simulink model "Fig_7_8__extflc"  (R2024a)
settings: Solver=VariableStepAuto  StartTime=0.0  StopTime=1  RelTol=1e-3
undefined symbols (not defined in the file): gcbh, Ion, Lithium, sps_rtmsupport
libraries: spsSeriesRLCBranchLib x11, spsThreePhaseVIMeasurementLib x5, slpidlib x5, spsIGBTDiodeLib x4, spsVoltageMeasurementLib x4, spsThreePhaseSeriesRLCBranchLib x4, spsUniversalBridgeLib x3, spsPWMGeneratorDCDCLib x3, spsBreakerLib x3, spsDiodeLib x2, spsabctodq0Lib x2, spsCurrentMeasurementLib x2
(part 2 of 2)

== system Fig_7_8__extflc/EVFCS/Battery charging controller ==
  note: Constant current battery charger control
  Add : Sum  Inputs=+-
  Add1 : Sum  Inputs=+-
  PID Controller1 : slpidlib/PID Controller  Controller=PI  Form=Parallel  TimeDomain=Discrete-time  UseExternalTs=off  SampleTime=-1  IntegratorMethod=Forward Euler  FilterMethod=Forward Euler  ControllerParametersSource=internal  P=5  I=0.0005  UseKiTs=off  D=0  UseExternalDerivativeSource=off  N=100  UseFilter=on  TunerSelectOption=Frequency Response Based  InitialConditionSource=internal  InitialConditionForIntegrator=0  InitialConditionForFilter=0  DifferentiatorICPrevScaledInput=0  ExternalReset=none  TrackingMode=off  Kt=1  LimitOutput=off  SatLimitsSource=internal  UpperSaturationLimit=1  LowerSaturationLimit=0  LinearizeAsGain=on  AntiWindupMode=none  Kb=1  LimitIntegrator=off  UpperIntegratorSaturationLimit=inf  LowerIntegratorSaturationLimit=-inf  POutMin=[]  POutMax=[]  IOutMin=[]  IOutMax=[]  DOutMin=[]  DOutMax=[]  NOutMin=[]  NOutMax=[]  SumOutMin=[]  SumOutMax=[]  SaturationOutMin=[]  SaturationOutMax=[]  PParamMin=[]  PParamMax=[]  IParamMin=[]  IParamMax=[]  DParamMin=[]  DParamMax=[]  NParamMin=[]  NParamMax=[]  KbParamMin=[]  KbParamMax=[]  KtParamMin=[]  KtParamMax=[]  KbOutMin=[]  KbOutMax=[]  KtOutMin=[]  KtOutMax=[]  IntegratorOutMin=[]  IntegratorOutMax=[]  FilterOutMin=[]  FilterOutMax=[]  SumI1OutMin=[]  SumI1OutMax=[]  SumI2OutMin=[]  SumI2OutMax=[]  SumI3OutMin=[]  SumI3OutMax=[]  SumI4OutMin=[]  SumI4OutMax=[]  SumDOutMin=[]  SumDOutMax=[]  DifferentiatorOutMin=[]  DifferentiatorOutMax=[]  FilterDiffOutCoefMin=[]  FilterDiffOutCoefMax=[]  ReciprocalOutMin=[]  ReciprocalOutMax=[]  SumDenOutMin=[]  SumDenOutMax=[]  SumNumOutMin=[]  SumNumOutMax=[]  DivideOutMin=[]  DivideOutMax=[]  UdiffTsProdOutMin=[]  UdiffTsProdOutMax=[]  NTsProdOutMin=[]  NTsProdOutMax=[]  UintegralTsProdOutMin=[]  UintegralTsProdOutMax=[]  UngainTsProdOutMin=[]  UngainTsProdOutMax=[]  ClampingZeroOutDataTypeStr=Inherit: Inherit via back propagation  ClampingZeroOutMin=[]  ClampingZeroOutMax=[]  FilterDenConstantOutDataTypeStr=Inherit: Inherit via back propagation  FilterDenConstantOutMin=[]  FilterDenConstantOutMax=[]  PCopyOutDataTypeStr=Inherit: Inherit via back propagation  PCopyOutMin=[]  PCopyOutMax=[]  NCopyOutDataTypeStr=Inherit: Inherit via back propagation  NCopyOutMin=[]  NCopyOutMax=[]  IntegratorContinuousStateAttributes=''  IntegratorStateMustResolveToSignalObject=off  IntegratorRTWStateStorageClass=Auto  FilterContinuousStateAttributes=''  FilterStateMustResolveToSignalObject=off  FilterRTWStateStorageClass=Auto  ParallelPVariant=InternalParameters  IdealPVariant=Disabled  IVariant=InternalParameters  DVariant=Disabled  IntegratorVariant=Discrete  SatVariant=Disabled  AWVariant=Passthrough  PCopyVariant=Disabled  TRVariant=Disabled  FdbkBlocksVariant=Forward  IdealPFdbkVariant=Disabled  SatFdbkVariant=Disabled  DerivativeFilterVariant=Disabled  NVariant=Disabled  NCopyVariant=Disabled_SignalSpec  FilterICVariant=Disabled  IntegratorICVariant=InternalICs  ExternalResetVariant=Disabled  TRSumVariant=Passthrough  SumFdbkVariant=Disabled  SumVariant=Sum_PI  TsampFilterVariant=InternalTs  TsampNgainVariant=Passthrough  TsampIntegralVariant=Disabled_SignalSpec  ExternalSaturationOutDataTypeStr=Inherit: Same as second input  DerivativeSourceVariant=Disabled
  PID Controller2 : slpidlib/PID Controller  Controller=PI  Form=Parallel  TimeDomain=Discrete-time  UseExternalTs=off  SampleTime=-1  IntegratorMethod=Forward Euler  FilterMethod=Forward Euler  ControllerParametersSource=internal  P=-5  I=-0.0005  UseKiTs=off  D=0  UseExternalDerivativeSource=off  N=100  UseFilter=on  TunerSelectOption=Transfer Function Based (PID Tuner App)  InitialConditionSource=internal  InitialConditionForIntegrator=0  InitialConditionForFilter=0  DifferentiatorICPrevScaledInput=0  ExternalReset=none  TrackingMode=off  Kt=1  LimitOutput=off  SatLimitsSource=internal  UpperSaturationLimit=0  LowerSaturationLimit=-5  LinearizeAsGain=on  AntiWindupMode=none  Kb=1  LimitIntegrator=off  UpperIntegratorSaturationLimit=inf  LowerIntegratorSaturationLimit=-inf  POutMin=[]  POutMax=[]  IOutMin=[]  IOutMax=[]  DOutMin=[]  DOutMax=[]  NOutMin=[]  NOutMax=[]  SumOutMin=[]  SumOutMax=[]  SaturationOutMin=[]  SaturationOutMax=[]  PParamMin=[]  PParamMax=[]  IParamMin=[]  IParamMax=[]  DParamMin=[]  DParamMax=[]  NParamMin=[]  NParamMax=[]  KbParamMin=[]  KbParamMax=[]  KtParamMin=[]  KtParamMax=[]  KbOutMin=[]  KbOutMax=[]  KtOutMin=[]  KtOutMax=[]  IntegratorOutMin=[]  IntegratorOutMax=[]  FilterOutMin=[]  FilterOutMax=[]  SumI1OutMin=[]  SumI1OutMax=[]  SumI2OutMin=[]  SumI2OutMax=[]  SumI3OutMin=[]  SumI3OutMax=[]  SumI4OutMin=[]  SumI4OutMax=[]  SumDOutMin=[]  SumDOutMax=[]  DifferentiatorOutMin=[]  DifferentiatorOutMax=[]  FilterDiffOutCoefMin=[]  FilterDiffOutCoefMax=[]  ReciprocalOutMin=[]  ReciprocalOutMax=[]  SumDenOutMin=[]  SumDenOutMax=[]  SumNumOutMin=[]  SumNumOutMax=[]  DivideOutMin=[]  DivideOutMax=[]  UdiffTsProdOutMin=[]  UdiffTsProdOutMax=[]  NTsProdOutMin=[]  NTsProdOutMax=[]  UintegralTsProdOutMin=[]  UintegralTsProdOutMax=[]  UngainTsProdOutMin=[]  UngainTsProdOutMax=[]  ClampingZeroOutDataTypeStr=Inherit: Inherit via back propagation  ClampingZeroOutMin=[]  ClampingZeroOutMax=[]  FilterDenConstantOutDataTypeStr=Inherit: Inherit via back propagation  FilterDenConstantOutMin=[]  FilterDenConstantOutMax=[]  PCopyOutDataTypeStr=Inherit: Inherit via back propagation  PCopyOutMin=[]  PCopyOutMax=[]  NCopyOutDataTypeStr=Inherit: Inherit via back propagation  NCopyOutMin=[]  NCopyOutMax=[]  IntegratorContinuousStateAttributes=''  IntegratorStateMustResolveToSignalObject=off  IntegratorRTWStateStorageClass=Auto  FilterContinuousStateAttributes=''  FilterStateMustResolveToSignalObject=off  FilterRTWStateStorageClass=Auto  ParallelPVariant=InternalParameters  IdealPVariant=Disabled  IVariant=InternalParameters  DVariant=Disabled  IntegratorVariant=Discrete  SatVariant=Disabled  AWVariant=Passthrough  PCopyVariant=Disabled  TRVariant=Disabled  FdbkBlocksVariant=Forward  IdealPFdbkVariant=Disabled  SatFdbkVariant=Disabled  DerivativeFilterVariant=Disabled  NVariant=Disabled  NCopyVariant=Disabled_SignalSpec  FilterICVariant=Disabled  IntegratorICVariant=InternalICs  ExternalResetVariant=Disabled  TRSumVariant=Passthrough  SumFdbkVariant=Disabled  SumVariant=Sum_PI  TsampFilterVariant=InternalTs  TsampNgainVariant=Passthrough  TsampIntegralVariant=Disabled_SignalSpec  ExternalSaturationOutDataTypeStr=Inherit: Same as second input  DerivativeSourceVariant=Disabled
  PWM Generator (DC-DC)1 : spsPWMGeneratorDCDCLib/PWM Generator (DC-DC)  Fsw=20e3  Ts=50e-6
  Vev_ref : Constant  Value=480
  G : Outport
  wires:
  PWM Generator (DC-DC)1/1 -> G/1
  Add/1 -> PID Controller2/1
  Vev_ref/1 -> Add/1
  [Vev] -> Add/2
  [Iev] -> Add1/2
  PID Controller2/1 -> Add1/1
  Add1/1 -> PID Controller1/1
  PID Controller1/1 -> PWM Generator (DC-DC)1/1

== system Fig_7_8__extflc/Dstatcom/Controller/FLC ==
  error : Inport
  Derivative : Derivative
  Fuzzy Logic Controller : fuzblock/Fuzzy Logic  Controller  FIS=flcabcdef  OutputSampleNumber=2  DataType=double  FuzzifiedInputs=off  RuleFiringStrengths=off  RuleOutputs=off  AggregatedOutputs=off  SimulateUsing=Interpreted execution  OutOfRangeInputValueMessage=none  NoRuleFiredMessage=none  EmptyOutputFuzzySetMessage=none
  Mux : Mux  Inputs=2
  output : Outport
  wires:
  Fuzzy Logic Controller/1 -> output/1
  Mux/1 -> Fuzzy Logic Controller/1
  Derivative/1 -> Mux/2
  error/1 -> Derivative/1, Mux/1

== system Fig_7_8__extflc/Dstatcom/Controller/PI1 ==
  In1 : Inport
  Integrator : Integrator  LimitOutput=on  UpperSaturationLimit=500  LowerSaturationLimit=-500
  Ki : Gain  Gain=1200
  Kp : Gain  Gain=800
  Sum8 : Sum  Inputs=|++
  Out1 : Outport
  wires:
  Ki/1 -> Integrator/1
  Kp/1 -> Sum8/1
  Integrator/1 -> Sum8/2
  In1/1 -> Kp/1, Ki/1
  Sum8/1 -> Out1/1

== system Fig_7_8__extflc/Dstatcom/Controller/RYB - ab ==
  Ilr : Inport
  Ily : Inport  Port=2
  Ilb : Inport  Port=3
  Demux : Demux  Outputs=2
  Gain : Gain  Gain=[1 -0.5 -0.5;0 0.866 -0.866]  Multiplication=Matrix(K*u)
  Mux : Mux  Inputs=3
  a : Outport
  b : Outport  Port=2
  wires:
  Demux/1 -> a/1
  Mux/1 -> Gain/1
  Demux/2 -> b/1
  Ilr/1 -> Mux/1
  Ilb/1 -> Mux/3
  Gain/1 -> Demux/1
  Ily/1 -> Mux/2

== system Fig_7_8__extflc/Dstatcom/Controller/RYB - ab1 ==
  Vgr : Inport
  Vgy : Inport  Port=2
  Vgb : Inport  Port=3
  Demux : Demux  Outputs=2
  Gain : Gain  Gain=[1 -0.5 -0.5;0 0.866 -0.866]  Multiplication=Matrix(K*u)
  Mux : Mux  Inputs=3
  Scope : Scope  NumInputPorts=2
  Va : Outport
  Vb : Outport  Port=2
  wires:
  Demux/1 -> Va/1
  Mux/1 -> Scope/2, Gain/1
  Demux/2 -> Scope/1, Vb/1
  Vgr/1 -> Mux/1
  Vgb/1 -> Mux/3
  Gain/1 -> Demux/1
  Vgy/1 -> Mux/2

== system Fig_7_8__extflc/Dstatcom/Controller/RYB - ab2 ==
  Isr : Inport
  Isy : Inport  Port=2
  Isb : Inport  Port=3
  Demux : Demux  Outputs=2
  Gain : Gain  Gain=[1 -0.5 -0.5;0 0.866 -0.866]  Multiplication=Matrix(K*u)
  Mux : Mux  Inputs=3
  Scope : Scope  NumInputPorts=2
  a : Outport
  b : Outport  Port=2
  wires:
  Demux/1 -> a/1
  Mux/1 -> Scope/2, Gain/1
  Demux/2 -> b/1
  Isr/1 -> Mux/1
  Isb/1 -> Mux/3
  Isy/1 -> Mux/2
  Gain/1 -> Scope/1, Demux/1

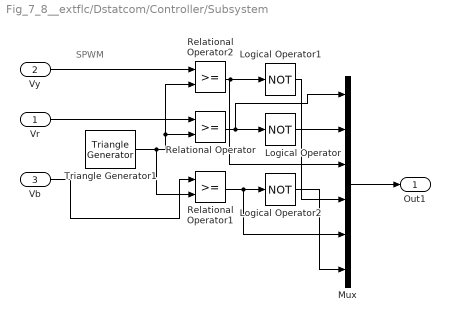
== system Fig_7_8__extflc/Dstatcom/Controller/Subsystem ==
  note: SPWM
  Vr : Inport
  Vy : Inport  Port=2
  Vb : Inport  Port=3
  Logical Operator : Logic  Operator=NOT  IconShape=distinctive  AllPortsSameDT=off  OutDataTypeStr=boolean
  Logical Operator1 : Logic  Operator=NOT  IconShape=distinctive  AllPortsSameDT=off  OutDataTypeStr=boolean
  Logical Operator2 : Logic  Operator=NOT  IconShape=distinctive  AllPortsSameDT=off  OutDataTypeStr=boolean
  Mux : Mux  Inputs=6
  Relational Operator : RelationalOperator  OutDataTypeStr=boolean  InputSameDT=off
  Relational Operator1 : RelationalOperator  OutDataTypeStr=boolean  InputSameDT=off
  Relational Operator2 : RelationalOperator  OutDataTypeStr=boolean  InputSameDT=off
  Triangle Generator1 : spsTriangleGeneratorLib/Triangle Generator  Freq=20e3  Phase=90  Ts=0
  Out1 : Outport
  wires:
  Triangle Generator1/1 -> Relational Operator2/2, Relational Operator/2, Relational Operator1/2
  Relational Operator2/1 -> Mux/3, Logical Operator1/1
  Relational Operator/1 -> Mux/1, Logical Operator/1
  Relational Operator1/1 -> Mux/5, Logical Operator2/1
  Mux/1 -> Out1/1
  Vy/1 -> Relational Operator2/1
  Logical Operator2/1 -> Mux/6
  Logical Operator1/1 -> Mux/4
  Logical Operator/1 -> Mux/2
  Vr/1 -> Relational Operator/1
  Vb/1 -> Relational Operator1/1

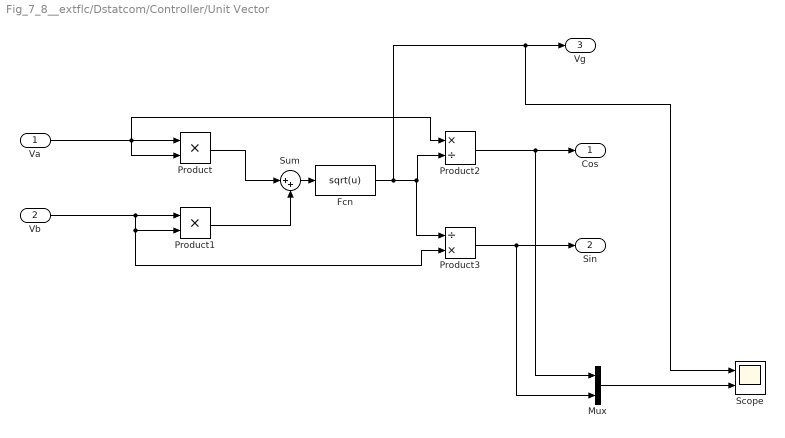
== system Fig_7_8__extflc/Dstatcom/Controller/Unit Vector ==
  Va : Inport
  Vb : Inport  Port=2
  Fcn : Fcn  Expr=sqrt(u)
  Mux : Mux  Inputs=2
  Product : Product
  Product1 : Product
  Product2 : Product  Inputs=*/
  Product3 : Product  Inputs=/*
  Scope : Scope  NumInputPorts=2
  Sum : Sum  Inputs=|++
  Cos : Outport
  Sin : Outport  Port=2
  Vg : Outport  Port=3
  wires:
  Sum/1 -> Fcn/1
  Va/1 -> Product2/1, Product/2, Product/1
  Vb/1 -> Product1/1, Product1/2, Product3/2
  Product/1 -> Sum/1
  Product1/1 -> Sum/2
  Product3/1 -> Mux/2, Sin/1
  Product2/1 -> Mux/1, Cos/1
  Fcn/1 -> Scope/1, Vg/1, Product3/1, Product2/2
  Mux/1 -> Scope/2

== system Fig_7_8__extflc/Dstatcom/Controller/ab - RYB ==
  a : Inport
  b : Inport  Port=2
  Demux : Demux  Outputs=3
  Gain : Gain  Gain=[1 0;-1/2 sqrt(3)/2;-1/2 -sqrt(3)/2]  Multiplication=Matrix(K*u)
  Mux : Mux  Inputs=2
  R : Outport
  Y : Outport  Port=2
  B : Outport  Port=3
  wires:
  b/1 -> Mux/2
  Gain/1 -> Demux/1
  a/1 -> Mux/1
  Demux/2 -> Y/1
  Mux/1 -> Gain/1
  Demux/1 -> R/1
  Demux/3 -> B/1

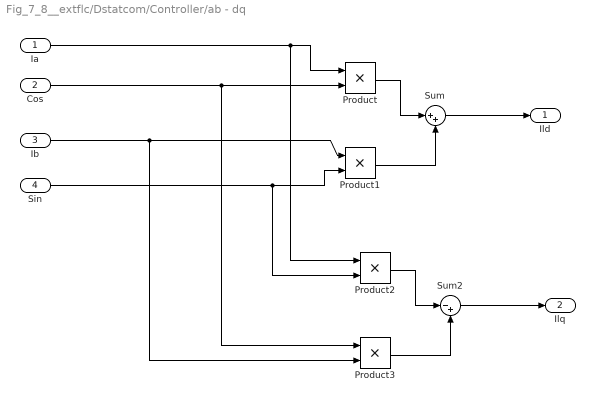
== system Fig_7_8__extflc/Dstatcom/Controller/ab - dq ==
  Ia : Inport
  Cos : Inport  Port=2
  Ib : Inport  Port=3
  Sin : Inport  Port=4
  Product{,1..3} (4 alike) : Product
  Sum : Sum  Inputs=|++
  Sum2 : Sum  Inputs=|-+
  Ild : Outport
  Ilq : Outport  Port=2
  wires:
  Product/1 -> Sum/1
  Sin/1 -> Product2/2, Product1/2
  Product1/1 -> Sum/2
  Ia/1 -> Product2/1, Product/1
  Sum/1 -> Ild/1
  Ib/1 -> Product3/2, Product1/1
  Product2/1 -> Sum2/1
  Product3/1 -> Sum2/2
  Sum2/1 -> Ilq/1
  Cos/1 -> Product3/1, Product/2

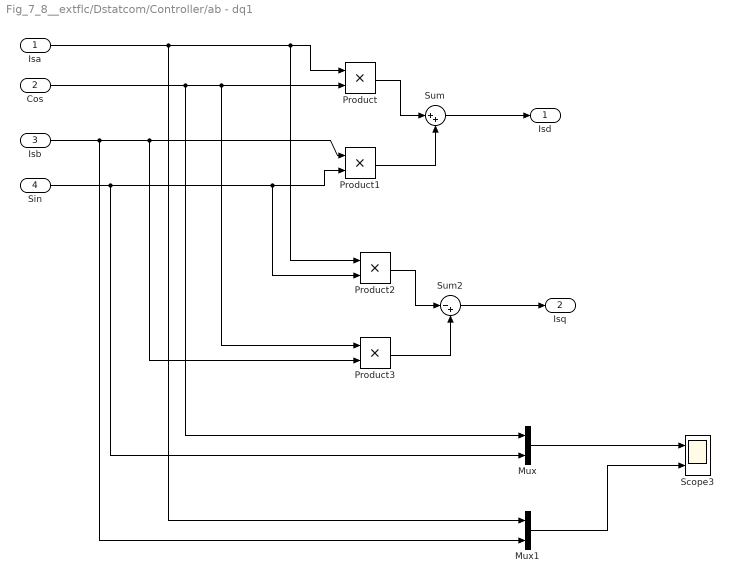
== system Fig_7_8__extflc/Dstatcom/Controller/ab - dq1 ==
  Isa : Inport
  Cos : Inport  Port=2
  Isb : Inport  Port=3
  Sin : Inport  Port=4
  Mux : Mux  Inputs=2
  Mux1 : Mux  Inputs=2
  Product{,1..3} (4 alike) : Product
  Scope3 : Scope  NumInputPorts=2
  Sum : Sum  Inputs=|++
  Sum2 : Sum  Inputs=|-+
  Isd : Outport
  Isq : Outport  Port=2
  wires:
  Product/1 -> Sum/1
  Sin/1 -> Mux/2, Product2/2, Product1/2
  Product1/1 -> Sum/2
  Isa/1 -> Mux1/1, Product2/1, Product/1
  Sum/1 -> Isd/1
  Isb/1 -> Mux1/2, Product3/2, Product1/1
  Product2/1 -> Sum2/1
  Product3/1 -> Sum2/2
  Sum2/1 -> Isq/1
  Cos/1 -> Mux/1, Product3/1, Product/2
  Mux/1 -> Scope3/1
  Mux1/1 -> Scope3/2

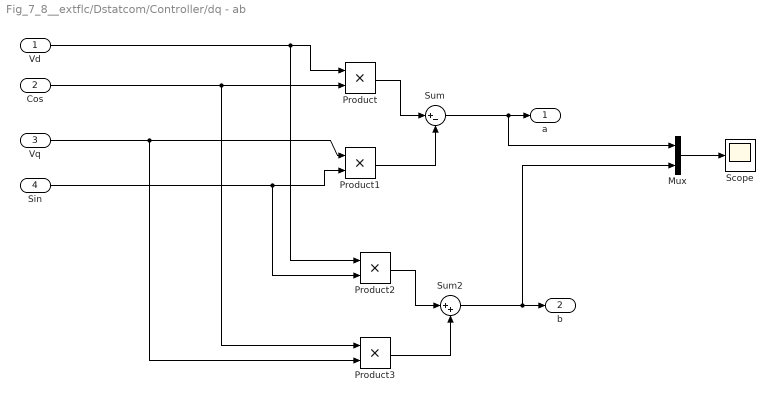
== system Fig_7_8__extflc/Dstatcom/Controller/dq - ab ==
  Vd : Inport
  Cos : Inport  Port=2
  Vq : Inport  Port=3
  Sin : Inport  Port=4
  Mux : Mux  Inputs=2
  Product{,1..3} (4 alike) : Product
  Scope : Scope
  Sum : Sum  Inputs=|+-
  Sum2 : Sum  Inputs=|++
  a : Outport
  b : Outport  Port=2
  wires:
  Cos/1 -> Product/2, Product3/1
  Sum2/1 -> Mux/2, b/1
  Product3/1 -> Sum2/2
  Product2/1 -> Sum2/1
  Vq/1 -> Product1/1, Product3/2
  Sum/1 -> Mux/1, a/1
  Vd/1 -> Product/1, Product2/1
  Product1/1 -> Sum/2
  Sin/1 -> Product1/2, Product2/2
  Product/1 -> Sum/1
  Mux/1 -> Scope/1

== system Fig_7_8__extflc/Dstatcom/D_Statcom/Subsystem ==
  Breaker : spsBreakerLib/Breaker  InitialState=1  SwitchingTimes="[1/60  5/60]"  External=on  BreakerResistance=0.01  SnubberResistance=1e6  SnubberCapacitance=inf  Measurements=None  MoreParameters=on  NoBreakLoop=off
  DC Voltage Source : spsDCVoltageSourceLib/DC Voltage Source  Amplitude=730  Measurements=None
  Series RLC Branch2 : spsSeriesRLCBranchLib/Series RLC Branch  LConnTagsString=__new0  RConnTagsString=__new0  BranchType=R  Resistance=0.001  Inductance=1e-3  SetiL0=off  InitialCurrent=0  Capacitance=1000e-6  Setx0=off  InitialVoltage=0  Measurements=None
  + : PMIOPort  Side=Left
  - : PMIOPort  Port=2  Side=Right
  wires:
  [T24_2155_1229794295581] -> Breaker/1
  connections:
  DC Voltage Source/RConn1 -- Series RLC Branch2/RConn1
  DC Voltage Source/LConn1 -- -/RConn1
  Breaker/LConn1 -- +/RConn1
  Breaker/RConn1 -- Series RLC Branch2/LConn1

== matlab function Fig_7_8__extflc/BOOST CONVERTER/PnO/PERTURB & OBSERVE ALGORITHM ==
  data: Vpv input; D output; Ipv input
function D = PnO(Vpv, Ipv)

persistent Dprev Pprev Vprev

if isempty(Dprev)
    Dprev = 0.7;
    Vprev = 145;
    Pprev = 1000;
end

deltaD = 125e-6

% Caluclate PV Power
Ppv = Vpv*Ipv

% Increase or decrease duty cycle based on conditions
if (Ppv-Pprev) ~= 0
    if (Ppv-Pprev) > 0
        if (Vpv-Vprev) > 0
            D = Dprev - deltaD;
        else
            D = Dprev + deltaD;
        end
    else
        if (Vpv - Vprev) > 0
            D = Dprev + deltaD;
        else
            D = Dprev - deltaD;
        end
    end
else
    D = Dprev;
end

% Update interval values
Dprev = D;
Vprev = Vpv;
Pprev = Ppv;

== matlab function Fig_7_8__extflc/BOOST CONVERTER1/PnO/PERTURB & OBSERVE ALGORITHM ==
  data: Vpv input; D output; Ipv input
function D = PnO(Vpv, Ipv)

persistent Dprev Pprev Vprev

if isempty(Dprev)
    Dprev = 0.7;
    Vprev = 145;
    Pprev = 1000;
end

deltaD = 125e-6

% Caluclate PV Power
Ppv = Vpv*Ipv

% Increase or decrease duty cycle based on conditions
if (Ppv-Pprev) ~= 0
    if (Ppv-Pprev) > 0
        if (Vpv-Vprev) > 0
            D = Dprev - deltaD;
        else
            D = Dprev + deltaD;
        end
    else
        if (Vpv - Vprev) > 0
            D = Dprev + deltaD;
        else
            D = Dprev - deltaD;
        end
    end
else
    D = Dprev;
end

% Update interval values
Dprev = D;
Vprev = Vpv;
Pprev = Ppv;
